simulink model "CPG"  (R2015a)
settings: Solver=ode8  StartTime=0.0  StopTime=20  FixedStep=0.001  RelTol=1e-3
values from neighbouring files (symbols this model uses):
  alpha = 1    [gaitGeneration.m]
  mu = 1    [gaitGeneration.m]    (also in path_planning.m = 0.7)
  omega = 1    [gaitGeneration.m]
  tau = 1    [gaitGeneration.m]
Description:
  | Central pattern generator for gaits
settings Model: Creator=marki  LastModifiedBy=marki

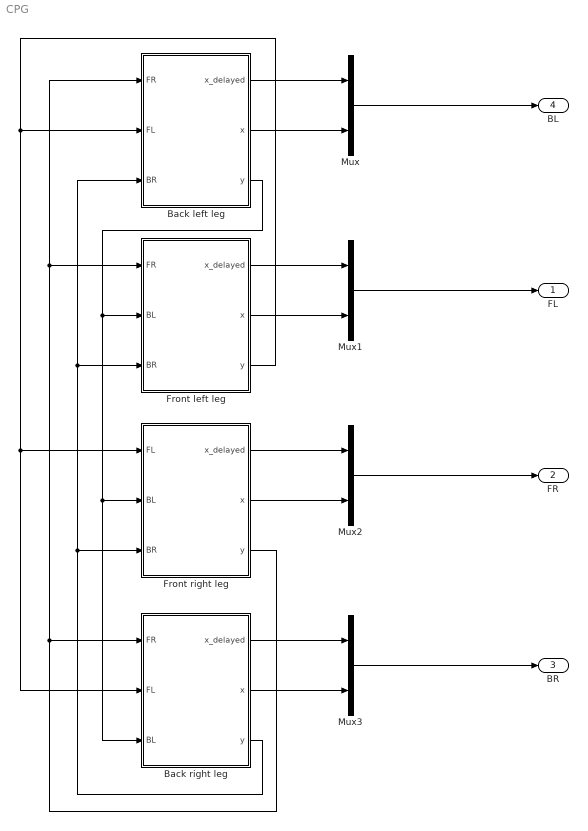
== system CPG ==
  Back left leg : Subsystem
  Back right leg : Subsystem
  Front left leg : Subsystem
  Front right leg : Subsystem
  Mux{,1..3} (4 alike) : Mux  Inputs=2
  FL : Outport
  FR : Outport  Port=2
  BR : Outport  Port=3
  BL : Outport  Port=4
  wires:
  Back left leg/3(y) -> Front left leg/2(BL), Front right leg/2(BL), Back right leg/3(BL)
  Back right leg/3(y) -> Front right leg/3(BR), Front left leg/3(BR), Back left leg/3(BR)
  Front right leg/3(y) -> Back left leg/1(FR), Front left leg/1(FR), Back right leg/1(FR)
  Front left leg/3(y) -> Back left leg/2(FL), Back right leg/2(FL), Front right leg/1(FL)
  Mux/1 -> BL/1
  Back left leg/1(x_delayed) -> Mux/1
  Back left leg/2(x) -> Mux/2
  Front left leg/1(x_delayed) -> Mux1/1
  Front left leg/2(x) -> Mux1/2
  Mux2/1 -> FR/1
  Front right leg/1(x_delayed) -> Mux2/1
  Front right leg/2(x) -> Mux2/2
  Back right leg/1(x_delayed) -> Mux3/1
  Back right leg/2(x) -> Mux3/2
  Mux1/1 -> FL/1
  Mux3/1 -> BR/1

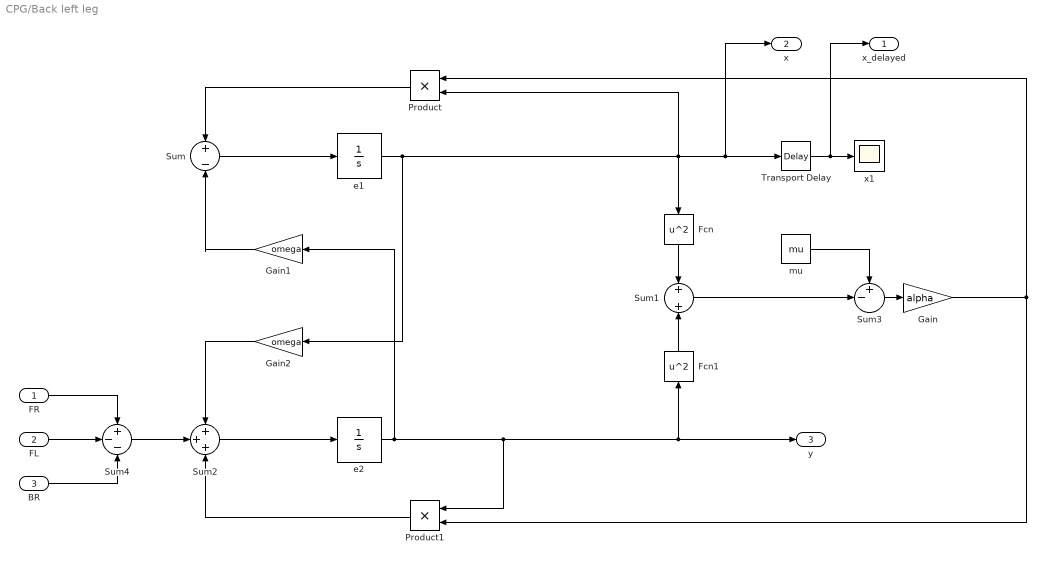
== system CPG/Back left leg ==
  FR : Inport
  FL : Inport  Port=2
  BR : Inport  Port=3
  Fcn : Fcn  Expr=u^2
  Fcn1 : Fcn  Expr=u^2
  Gain : Gain  Gain=alpha
  Gain1 : Gain  Gain=omega
  Gain2 : Gain  Gain=omega
  Product : Product
  Product1 : Product
  Sum : Sum  Inputs=+-
  Sum1 : Sum
  Sum2 : Sum  Inputs=+++
  Sum3 : Sum  Inputs=+-|
  Sum4 : Sum  Inputs=+--
  Transport Delay : TransportDelay  DelayTime=tau
  e1 : Integrator
  e2 : Integrator
  mu : Constant  Value=mu
  x1 : Scope
      settings: SaveName=ScopeData2
  x_delayed : Outport
  x : Outport  Port=2
  y : Outport  Port=3
  wires:
  Transport Delay/1 -> x_delayed/1, x1/1
  Sum4/1 -> Sum2/2
  Fcn1/1 -> Sum1/2
  Sum3/1 -> Gain/1
  Sum1/1 -> Sum3/2
  Gain1/1 -> Sum/2
  BR/1 -> Sum4/3
  FL/1 -> Sum4/2
  mu/1 -> Sum3/1
  Product1/1 -> Sum2/3
  Sum/1 -> e1/1
  e1/1 -> Gain2/1, Product/2, x/1, Transport Delay/1, Fcn/1
  Product/1 -> Sum/1
  Fcn/1 -> Sum1/1
  Sum2/1 -> e2/1
  FR/1 -> Sum4/1
  e2/1 -> y/1, Fcn1/1, Product1/1, Gain1/1
  Gain/1 -> Product/1, Product1/2
  Gain2/1 -> Sum2/1

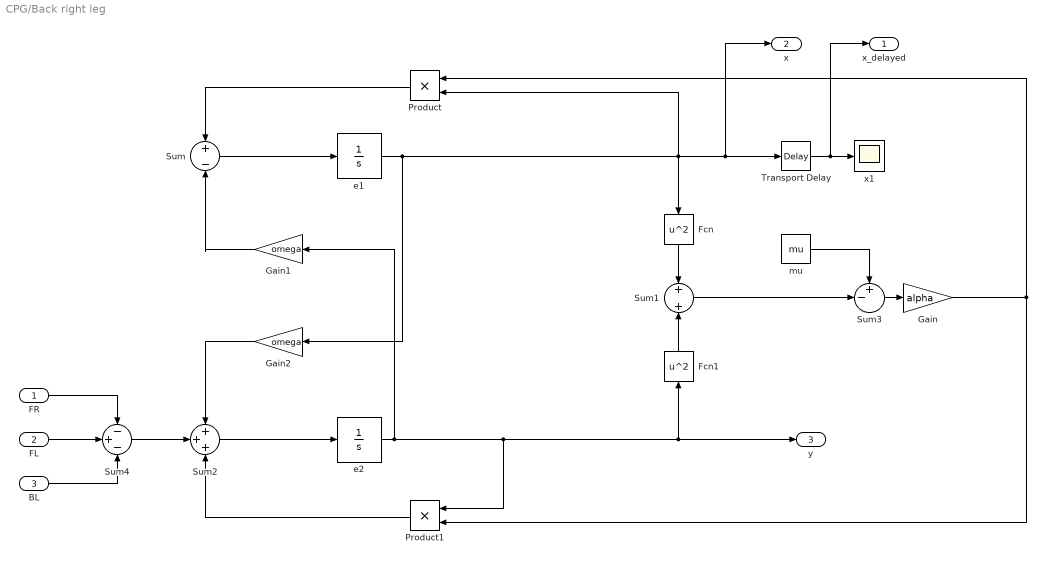
== system CPG/Back right leg ==
  FR : Inport
  FL : Inport  Port=2
  BL : Inport  Port=3
  Fcn : Fcn  Expr=u^2
  Fcn1 : Fcn  Expr=u^2
  Gain : Gain  Gain=alpha
  Gain1 : Gain  Gain=omega
  Gain2 : Gain  Gain=omega
  Product : Product
  Product1 : Product
  Sum : Sum  Inputs=+-
  Sum1 : Sum
  Sum2 : Sum  Inputs=+++
  Sum3 : Sum  Inputs=+-|
  Sum4 : Sum  Inputs=-+-
  Transport Delay : TransportDelay  DelayTime=tau
  e1 : Integrator
  e2 : Integrator
  mu : Constant  Value=mu
  x1 : Scope
      settings: SaveName=ScopeData2
  x_delayed : Outport
  x : Outport  Port=2
  y : Outport  Port=3
  wires:
  Transport Delay/1 -> x_delayed/1, x1/1
  Fcn1/1 -> Sum1/2
  Sum3/1 -> Gain/1
  Sum1/1 -> Sum3/2
  Gain1/1 -> Sum/2
  BL/1 -> Sum4/3
  FL/1 -> Sum4/2
  mu/1 -> Sum3/1
  Product1/1 -> Sum2/3
  Sum/1 -> e1/1
  e1/1 -> Gain2/1, Product/2, x/1, Transport Delay/1, Fcn/1
  Product/1 -> Sum/1
  Fcn/1 -> Sum1/1
  Sum2/1 -> e2/1
  FR/1 -> Sum4/1
  e2/1 -> y/1, Fcn1/1, Product1/1, Gain1/1
  Gain/1 -> Product/1, Product1/2
  Gain2/1 -> Sum2/1
  Sum4/1 -> Sum2/2

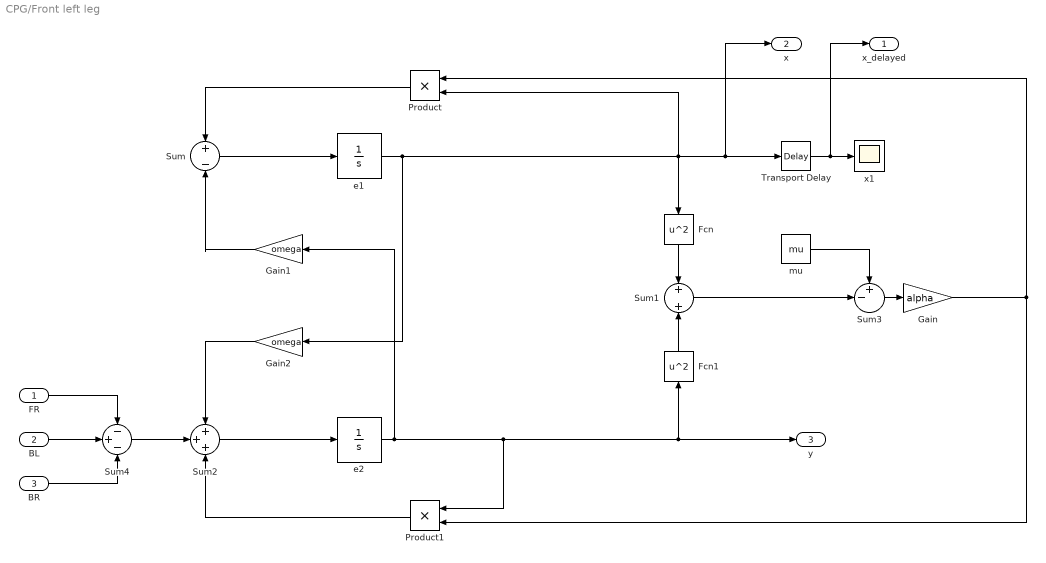
== system CPG/Front left leg ==
  FR : Inport
  BL : Inport  Port=2
  BR : Inport  Port=3
  Fcn : Fcn  Expr=u^2
  Fcn1 : Fcn  Expr=u^2
  Gain : Gain  Gain=alpha
  Gain1 : Gain  Gain=omega
  Gain2 : Gain  Gain=omega
  Product : Product
  Product1 : Product
  Sum : Sum  Inputs=+-
  Sum1 : Sum
  Sum2 : Sum  Inputs=+++
  Sum3 : Sum  Inputs=+-|
  Sum4 : Sum  Inputs=-+-
  Transport Delay : TransportDelay  DelayTime=tau
  e1 : Integrator
  e2 : Integrator  InitialCondition=1
  mu : Constant  Value=mu
  x1 : Scope
      settings: SaveName=ScopeData2
  x_delayed : Outport
  x : Outport  Port=2
  y : Outport  Port=3
  wires:
  Transport Delay/1 -> x_delayed/1, x1/1
  Sum4/1 -> Sum2/2
  Fcn1/1 -> Sum1/2
  Sum3/1 -> Gain/1
  Sum1/1 -> Sum3/2
  Gain1/1 -> Sum/2
  BR/1 -> Sum4/3
  BL/1 -> Sum4/2
  mu/1 -> Sum3/1
  Product1/1 -> Sum2/3
  Sum/1 -> e1/1
  e1/1 -> Gain2/1, Product/2, x/1, Transport Delay/1, Fcn/1
  Product/1 -> Sum/1
  Fcn/1 -> Sum1/1
  Sum2/1 -> e2/1
  FR/1 -> Sum4/1
  e2/1 -> y/1, Fcn1/1, Product1/1, Gain1/1
  Gain/1 -> Product/1, Product1/2
  Gain2/1 -> Sum2/1

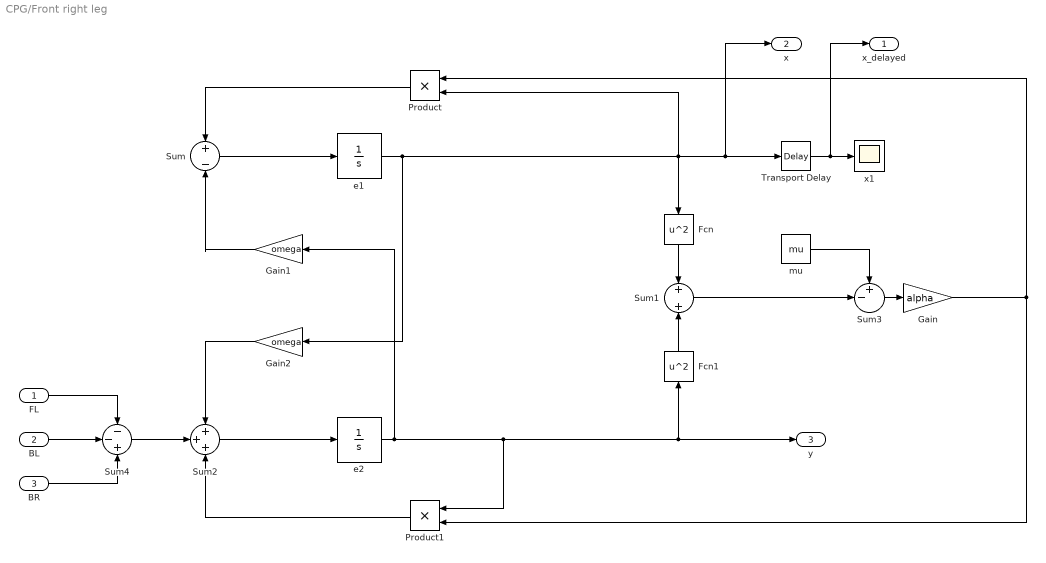
== system CPG/Front right leg ==
  FL : Inport
  BL : Inport  Port=2
  BR : Inport  Port=3
  Fcn : Fcn  Expr=u^2
  Fcn1 : Fcn  Expr=u^2
  Gain : Gain  Gain=alpha
  Gain1 : Gain  Gain=omega
  Gain2 : Gain  Gain=omega
  Product : Product
  Product1 : Product
  Sum : Sum  Inputs=+-
  Sum1 : Sum
  Sum2 : Sum  Inputs=+++
  Sum3 : Sum  Inputs=+-|
  Sum4 : Sum  Inputs=--+
  Transport Delay : TransportDelay  DelayTime=tau
  e1 : Integrator
  e2 : Integrator
  mu : Constant  Value=mu
  x1 : Scope
      settings: SaveName=ScopeData2
  x_delayed : Outport
  x : Outport  Port=2
  y : Outport  Port=3
  wires:
  Transport Delay/1 -> x_delayed/1, x1/1
  Sum4/1 -> Sum2/2
  Fcn1/1 -> Sum1/2
  Sum3/1 -> Gain/1
  Sum1/1 -> Sum3/2
  Gain1/1 -> Sum/2
  BR/1 -> Sum4/3
  BL/1 -> Sum4/2
  mu/1 -> Sum3/1
  Product1/1 -> Sum2/3
  Sum/1 -> e1/1
  e1/1 -> Gain2/1, Product/2, x/1, Transport Delay/1, Fcn/1
  Product/1 -> Sum/1
  Fcn/1 -> Sum1/1
  Sum2/1 -> e2/1
  FL/1 -> Sum4/1
  e2/1 -> y/1, Fcn1/1, Product1/1, Gain1/1
  Gain/1 -> Product/1, Product1/2
  Gain2/1 -> Sum2/1
